simulink model "ADAS_System"  (R2025b)
settings: Solver=VariableStepAuto  StartTime=0.0  StopTime=10.0  RelTol=1e-3
values from neighbouring files (symbols this model uses):
  a_ego = 2    [init_ADAS.m]
  a_max = 10    [init_ADAS.m]
  d_init = 160    [init_ADAS.m]
  fs = 100    [init_ADAS.m]
  v_ego = 40    [init_ADAS.m]
  v_lead = 25    [init_ADAS.m]
libraries: simulink x6
settings Model: Creator=szymo

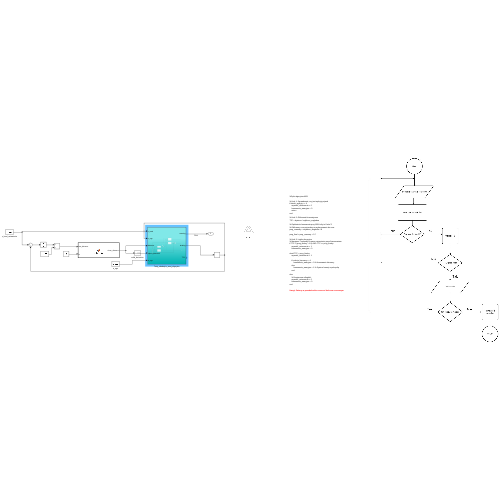
[thumbnail: Simulink's stored preview of the top-level diagram]
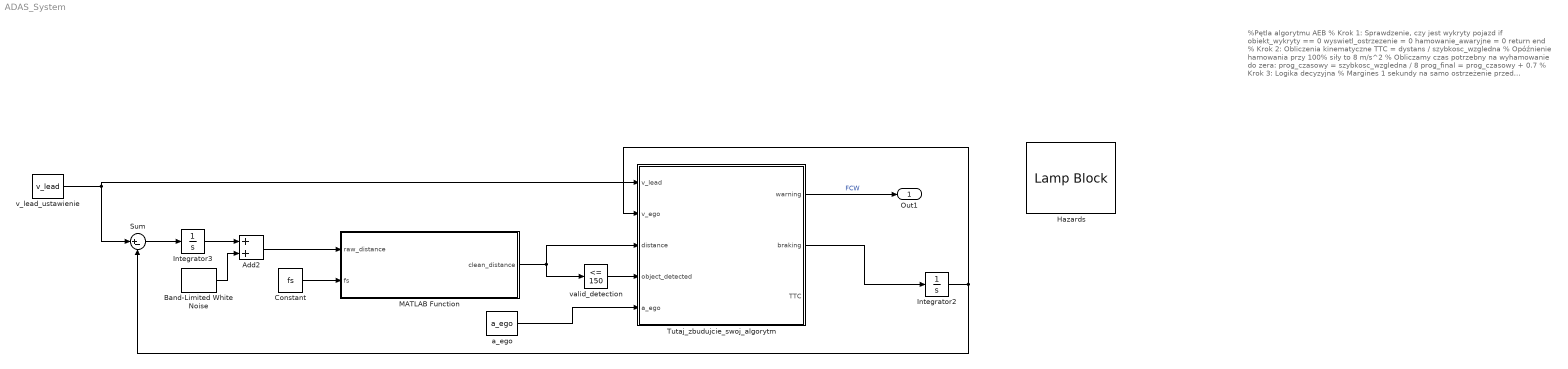
== system ADAS_System ==
  note: %Pętla algorytmu AEB
      |
      | % Krok 1: Sprawdzenie, czy jest wykryty pojazd
      | if obiekt_wykryty == 0
      | wyswietl_ostrzezenie = 0
      | hamowanie_awaryjne = 0
      | return
      | end
      |
      | % Krok 2: Obliczenia kinematyczne
      | TTC = dystans / szybkosc_wzgledna
      |
      | % Opóźnienie hamowania przy 100% siły to 8 m/s^2
      | % Obliczamy czas potrzebny na wyhamowanie do zera:
      | prog_czasowy = szybkosc_wzgledna / 8
      |
      | prog_final = prog_czasowy + 0.7
      |
      | % Krok 3: Logika decyzyjna
      | % Margines 1 sekundy na samo ostrzeżenie przed hamowaniem
      | if TTC < (prog_finalny + 1.0) AND TTC >= prog_finalny
      | wyswietl_ostrzezenie = 1
      | hamowanie_awaryjne = 0
      |
      | elseif TTC < prog_finalny
      | wyswietl_ostrzezenie = 1
      |
      | if reakcja_kierowcy == 1
      | hamowanie_awaryjne = 0 % Hamowanie kierowcy
      | else
      | hamowanie_awaryjne = 1 % System hamuje z pełną siłą
      | end
      |
      | else
      | % Bezpieczna odległość
      | wyswietl_ostrzezenie = 0
      | hamowanie_awaryjne = 0
      | end
      |
      | Uwagi: Zmiany w pseudokodzie oznaczać kolorem czerwonym
  Add2 : Sum
  Band-Limited White Noise : simulink/Sources/Band-Limited White Noise  Cov=[0.1]  Ts=0.1  seed=[23341]
  Constant : Constant  Value=fs
  Hazards : LampBlock  LabelPosition=Bottom  DefaultColor=[192.0, 192.0, 192.0]  Icon=Hazards
  Integrator2 : Integrator  InitialCondition=v_ego
  Integrator3 : Integrator  InitialCondition=d_init
  MATLAB Function : MATLAB Function  TreatAsAtomicUnit=on
  Sum : Sum  Inputs=|+-
  Tutaj_zbudujcie_swoj_algorytm : Subsystem
  a_ego : Constant  Value=a_ego  OutMin=[-8]  OutMax=[a_max]
  v_lead_ustawienie : Constant  Value=v_lead
  valid_detection : simulink/Logic and Bit Operations/Compare To Constant  relop=<=  const=150  OutDataTypeStr=boolean
  Out1 : Outport
  wires:
  Band-Limited White Noise/1 -> Add2/2
  Add2/1 -> MATLAB Function/1(raw_distance)
  Constant/1 -> MATLAB Function/2(fs)
  Tutaj_zbudujcie_swoj_algorytm/2(braking) -> Integrator2/1
  Integrator2/1 -> Tutaj_zbudujcie_swoj_algorytm/2(v_ego), Sum/2
  v_lead_ustawienie/1 -> Sum/1, Tutaj_zbudujcie_swoj_algorytm/1(v_lead)
  Sum/1 -> Integrator3/1
  Integrator3/1 -> Add2/1
  MATLAB Function/1(clean_distance) -> valid_detection/1, Tutaj_zbudujcie_swoj_algorytm/3(distance)
  valid_detection/1 -> Tutaj_zbudujcie_swoj_algorytm/4(object_detected)
  Tutaj_zbudujcie_swoj_algorytm/1(warning) -> Out1/1  "FCW"
  a_ego/1 -> Tutaj_zbudujcie_swoj_algorytm/5(a_ego)

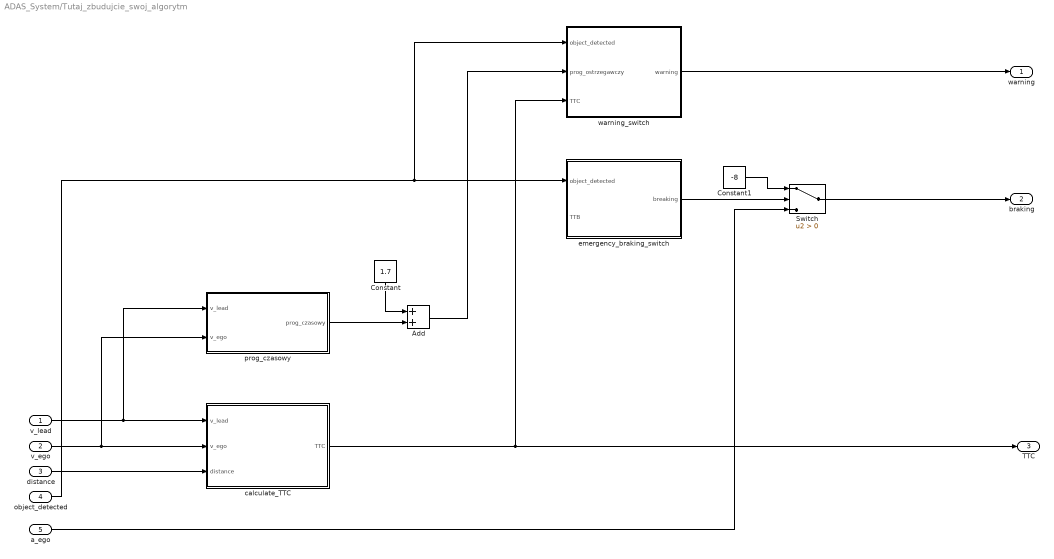
== system ADAS_System/Tutaj_zbudujcie_swoj_algorytm ==
  v_lead : Inport
  v_ego : Inport  Port=2
  distance : Inport  Port=3
  object_detected : Inport  Port=4
  a_ego : Inport  Port=5
  Add : Sum
  Constant : Constant  Value=1.7
  Constant1 : Constant  Value=-8
  Switch : Switch  Criteria=u2 > Threshold  SaturateOnIntegerOverflow=off  InputSameDT=off
  calculate_TTC : Subsystem
  emergency_braking_switch : Subsystem
  prog_czasowy : Subsystem
  warning_switch : Subsystem
  warning : Outport
  braking : Outport  Port=2
  "TTC " : Outport  Port=3
  wires:
  calculate_TTC/1(TTC) -> warning_switch/3(TTC), "TTC "/1
  warning_switch/1(warning) -> warning/1
  distance/1 -> calculate_TTC/3(distance)
  v_ego/1 -> prog_czasowy/2(v_ego), calculate_TTC/2(v_ego)
  object_detected/1 -> warning_switch/1(object_detected), emergency_braking_switch/1(object_detected)
  v_lead/1 -> prog_czasowy/1(v_lead), calculate_TTC/1(v_lead)
  prog_czasowy/1(prog_czasowy) -> Add/2
  Add/1 -> warning_switch/2(prog_ostrzegawczy)
  Constant/1 -> Add/1
  a_ego/1 -> Switch/3
  emergency_braking_switch/1(breaking) -> Switch/2
  Constant1/1 -> Switch/1
  Switch/1 -> braking/1

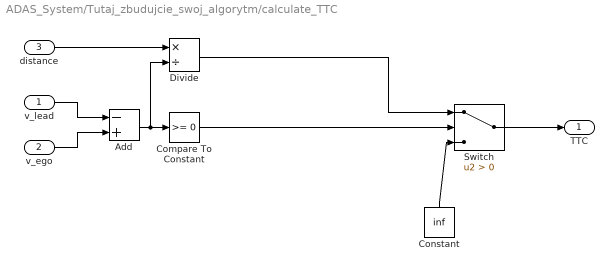
== system ADAS_System/Tutaj_zbudujcie_swoj_algorytm/calculate_TTC ==
  v_lead : Inport
  v_ego : Inport  Port=2
  distance : Inport  Port=3
  Add : Sum  Inputs=-+
  Compare To Constant : simulink/Logic and Bit Operations/Compare To Constant  relop=>=  const=0  OutDataTypeStr=boolean
  Constant : Constant  Value=inf
  Divide : Product  Inputs=*/
  Switch : Switch  Criteria=u2 > Threshold  SaturateOnIntegerOverflow=off  InputSameDT=off
  TTC : Outport
  wires:
  v_lead/1 -> Add/1
  v_ego/1 -> Add/2
  Add/1 -> Compare To Constant/1, Divide/2
  distance/1 -> Divide/1
  Switch/1 -> TTC/1
  Divide/1 -> Switch/1
  Constant/1 -> Switch/3
  Compare To Constant/1 -> Switch/2

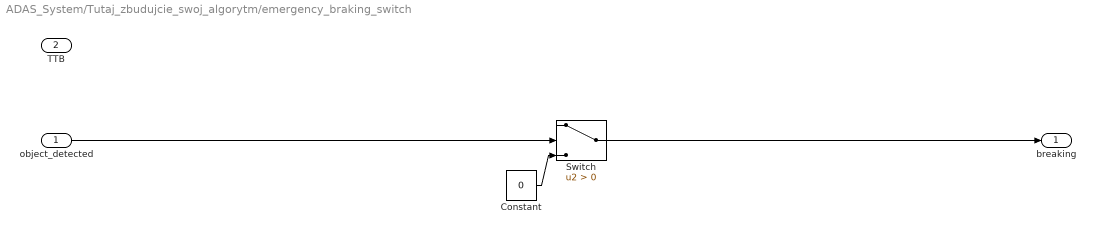
== system ADAS_System/Tutaj_zbudujcie_swoj_algorytm/emergency_braking_switch ==
  object_detected : Inport
  TTB : Inport  Port=2
  Constant : Constant  Value=0
  Switch : Switch  Criteria=u2 > Threshold  SaturateOnIntegerOverflow=off  InputSameDT=off
  breaking : Outport
  wires:
  object_detected/1 -> Switch/2
  Switch/1 -> breaking/1
  Constant/1 -> Switch/3

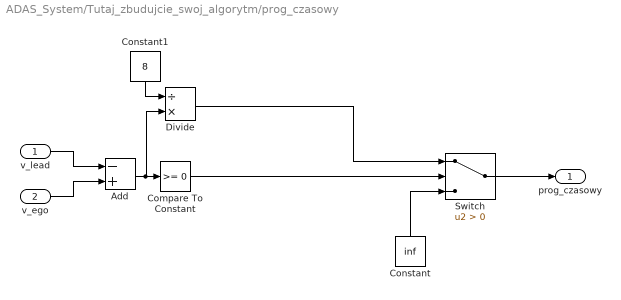
== system ADAS_System/Tutaj_zbudujcie_swoj_algorytm/prog_czasowy ==
  v_lead : Inport
  v_ego : Inport  Port=2
  Add : Sum  Inputs=-+
  Compare To Constant : simulink/Logic and Bit Operations/Compare To Constant  relop=>=  const=0  OutDataTypeStr=boolean
  Constant : Constant  Value=inf
  Constant1 : Constant  Value=8
  Divide : Product  Inputs=/*
  Switch : Switch  Criteria=u2 > Threshold  SaturateOnIntegerOverflow=off  InputSameDT=off
  prog_czasowy : Outport
  wires:
  Constant/1 -> Switch/3
  v_lead/1 -> Add/1
  v_ego/1 -> Add/2
  Switch/1 -> prog_czasowy/1
  Add/1 -> Divide/2, Compare To Constant/1
  Compare To Constant/1 -> Switch/2
  Divide/1 -> Switch/1
  Constant1/1 -> Divide/1

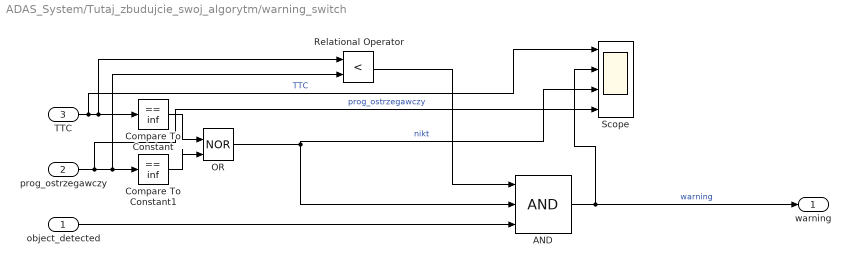
== system ADAS_System/Tutaj_zbudujcie_swoj_algorytm/warning_switch ==
  object_detected : Inport
  prog_ostrzegawczy : Inport  Port=2
  TTC : Inport  Port=3
  AND : Logic  Inputs=3  IconShape=distinctive  AllPortsSameDT=off  OutDataTypeStr=boolean
  Compare To Constant : simulink/Logic and Bit Operations/Compare To Constant  relop===  const=inf  OutDataTypeStr=boolean
  Compare To Constant1 : simulink/Logic and Bit Operations/Compare To Constant  relop===  const=inf  OutDataTypeStr=boolean
  OR : Logic  Operator=NOR  IconShape=distinctive  AllPortsSameDT=off  OutDataTypeStr=boolean
  Relational Operator : RelationalOperator  Operator=<  OutDataTypeStr=boolean  RndMeth=Simplest  InputSameDT=off
  Scope : Scope  NumInputPorts=4
      settings: ActiveDisplayYMinimum=-6.6250697146342548  ActiveDisplayYMaximum=21.353379825711041
  warning : Outport
  wires:
  AND/1 -> Scope/2, warning/1  "warning"
  Relational Operator/1 -> AND/1
  prog_ostrzegawczy/1 -> Scope/4, Relational Operator/2, Compare To Constant1/1  "prog_ostrzegawczy"
  TTC/1 -> Scope/1, Relational Operator/1, Compare To Constant/1  "TTC"
  Compare To Constant/1 -> OR/1
  Compare To Constant1/1 -> OR/2
  OR/1 -> AND/2, Scope/3  "nikt"
  object_detected/1 -> AND/3

== matlab function ADAS_System/MATLAB Function ==
  settings: updateMethod=DISCRETE
  data: raw_distance input; clean_distance output; fs input
function clean_distance = radar_filter(raw_distance, fs)
    persistent last_dist;
    
    % Inicjalizacja przy pierwszym kroku symulacji
    if isempty(last_dist)
        last_dist = raw_distance;
    end  
    
    % Obliczenie kroku czasu na podstawie częstotliwości próbkowania
    dt = 1 / fs; 
    
    tau = 0.02; 
    
    % Dynamiczne obliczenie wagi dla nowego pomiaru
    alpha = dt / (tau + dt); 
    
    % Filtracja: waga_nowego * nowy_pomiar + waga_starego * stary_pomiar
    clean_distance = alpha * raw_distance + (1 - alpha) * last_dist;
    
    % Zapisanie obecnej wartości na potrzeby kolejnego kroku
    last_dist = clean_distance;
end
